simulink model "lab5_sim"  (R2022b)
settings: Solver=VariableStepAuto  StartTime=0.0  StopTime=czas_symulacji  RelTol=1e-3
values from neighbouring files (symbols this model uses):
  dqg = 0.1*qgN    (= 1000)    [lab5_modyfikacja.m]    (also in lab6.m; lab7.m)
  dTzew = 0    [lab5_modyfikacja.m]    (also in lab6.m; lab7.m)
  L11 = [Cvp (Kcwp+Kcp)]    [lab5_modyfikacja.m]    (also in lab6.m = 0.004; lab7.m = 0.004)
  L12 = [Cvp*Kcw (Kcw*(Kcwp+Kcp)+Kcwp*Kcp)]    [lab5_modyfikacja.m]    (also in lab6.m = 0.003; lab7.m = 0.003)
  L21 = Kcwp    (= 80.4597701149)    [lab5_modyfikacja.m]
  L22 = [Kcp*Cvw (Kcw*Kcp + Kcp*Kcwp + Kcwp*Kcw)]    [lab5_modyfikacja.m]
  M = [Cvw*Cvp (Cvw*(Kcwp+Kcp)+Cvp*(Kcw+Kcwp)) Kcw*Kcwp+Kcw*Kcp+Kcwp*Kcp]    [lab5_modyfikacja.m]
  t0 = 1000    [lab5_modyfikacja.m]    (also in lab6.m; lab7.m)
  Tp0 = ((a*Kcw*Twew0)+Kcp*Tzew0)/(a*Kcw+Kcp)    [Lab2.m]    (also in lab5_modyfikacja.m; lab6.m = 0; lab7.m = 10)
  Twew0 = (qg(i)*(a*Kcw+Kcp)+Tzew0*(Kcw*(a*Kcw+Kcp)+(a*Kcw*Kcp)))/(Kcw*(a*Kcw+Kcp)+a*Kcw*Kcp)    [Lab2.m]    (also in lab5_modyfikacja.m = (qg0*(a*Kcw+Kcp)+Tzew0*(Kcw*(a*Kcw+Kcp)+(a*Kcw*Kcp)))/(Kcw*(; lab6.m = 0; lab7.m = 20)
settings Model: Creator=kubab  LastModifiedBy=kubab
settings DataIOCC: ReturnWorkspaceOutputs=off

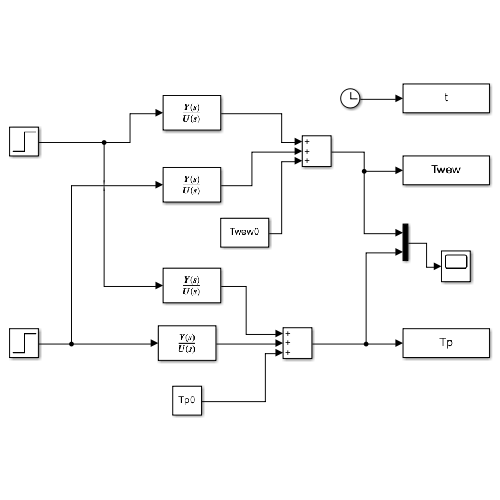
[thumbnail: Simulink's stored preview of the top-level diagram]
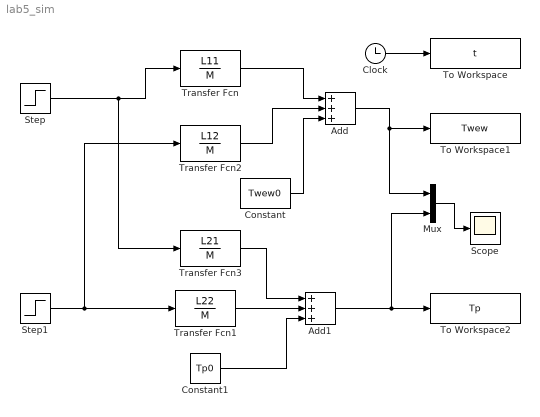
== system lab5_sim ==
  Add : Sum  Inputs=+++
  Add1 : Sum  Inputs=+++
  Clock : Clock
  Constant : Constant  Value=Twew0
  Constant1 : Constant  Value=Tp0
  Mux : Mux  Inputs=2
  Scope : Scope
  Step : Step  Time=t0  After=dqg  SampleTime=0
  Step1 : Step  Time=t0  After=dTzew  SampleTime=0
  To Workspace : ToWorkspace  VariableName=t  SaveFormat=Timeseries  SampleTime=-1
  To Workspace1 : ToWorkspace  VariableName=Twew  SampleTime=-1
  To Workspace2 : ToWorkspace  VariableName=Tp  SampleTime=-1
  Transfer Fcn : TransferFcn  Numerator=L11  Denominator=M
  Transfer Fcn1 : TransferFcn  Numerator=L22  Denominator=M
  Transfer Fcn2 : TransferFcn  Numerator=L12  Denominator=M
  Transfer Fcn3 : TransferFcn  Numerator=L21  Denominator=M
  wires:
  Step/1 -> Transfer Fcn3/1, Transfer Fcn/1
  Step1/1 -> Transfer Fcn2/1, Transfer Fcn1/1
  Transfer Fcn3/1 -> Add1/1
  Transfer Fcn1/1 -> Add1/2
  Transfer Fcn2/1 -> Add/2
  Transfer Fcn/1 -> Add/1
  Clock/1 -> To Workspace/1
  Add/1 -> Mux/1, To Workspace1/1
  Mux/1 -> Scope/1
  Add1/1 -> Mux/2, To Workspace2/1
  Constant/1 -> Add/3
  Constant1/1 -> Add1/3
